simulink model "WaypointGuidanceDemo_students_model"  (R2024a)
settings: Solver=VariableStepAuto  StartTime=0.0  StopTime=t_final  MaxStep=deltaTMax  RelTol=1e-3
values from neighbouring files (symbols this model uses):
  flightRoute = FlightRoute(waypoints_ENU, isClosed)    [MAIN_WaypointGuidanceDemo_students.m]
  waypointRadius = 100    [MAIN_WaypointGuidanceDemo_students.m]
undefined symbols (not defined in the file or in its folder): magnitude
libraries: aerolibutil x2, spsEdgeDetectorLib x1, vrlib x1
settings Model: Creator=Christopher  LastModifiedBy=chris
settings SolverCC: AlgebraicLoopSolver=TrustRegion
settings DataIOCC: ReturnWorkspaceOutputs=off
settings DebuggingCC: UnconnectedInputMsg=warning  UnconnectedOutputMsg=warning  UnconnectedLineMsg=warning  ArithmeticOperatorsInVariantConditions=warning
settings ModelReferenceCC: EnableRefExpFcnMdlSchedulingChecks=on
settings SFSimCC: CustomCodeUndefinedFunction=UseInterfaceOnly
settings RTWCC: GPUComputeCapability=3.5  DLArmComputeVersion=19.05

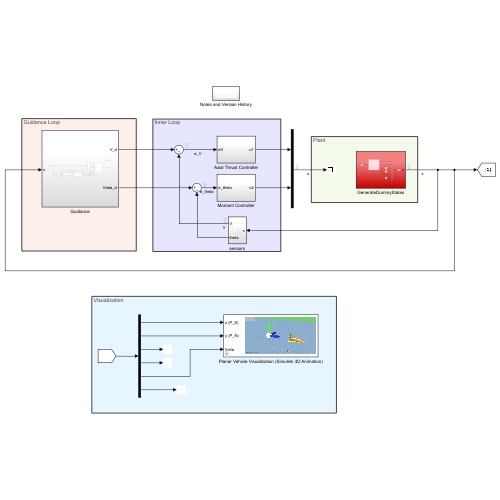
[thumbnail: Simulink's stored preview of the top-level diagram]
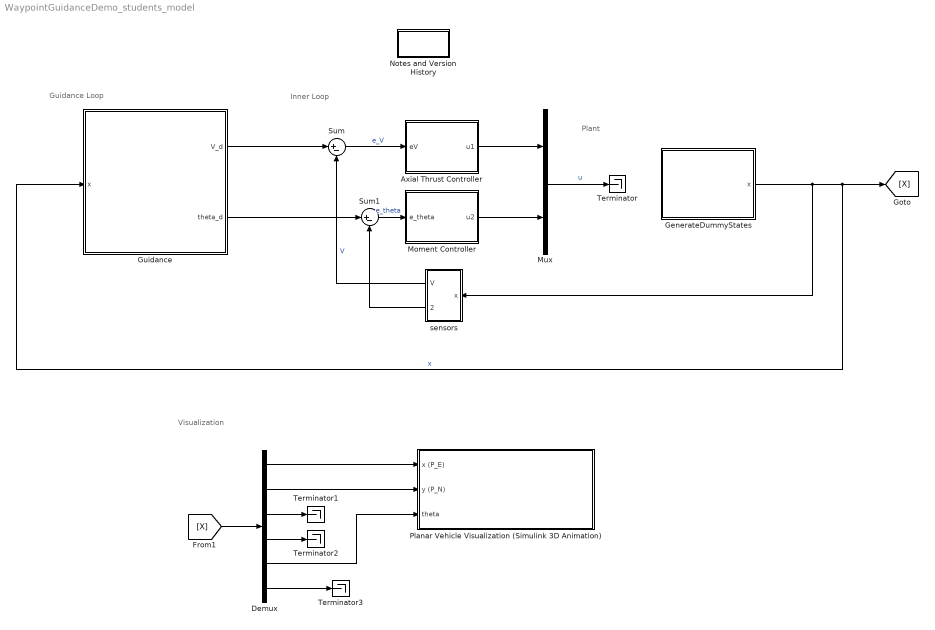
== system WaypointGuidanceDemo_students_model ==
  note: Plant
  note: Visualization
  note: Guidance Loop
  note: Inner Loop
  Axial Thrust Controller : Subsystem
  Demux : Demux  Outputs=6
  GenerateDummyStates : Subsystem
  Guidance : Subsystem
  Moment Controller : Subsystem
  Mux : Mux  Inputs=2
  Notes and Version History : Subsystem
  Planar Vehicle Visualization (Simulink 3D Animation) : Subsystem  mask{T_animate=1}
      mask prompts: T_animate "Time step for animation"
      mask help:
      | This is a visualization of the planar vehicle using the Simulink 3D Animation environment.
      |
      | Note: Simulink should open up the VRML sink and it should display the aircraft model in a separate window.  If this does not occur, you may need to look under the mask and through down through subsystems until you find the VR Sink block.  Double click on this block to open the animation window.
      |
      | Further note that Simulink may close the VRML sink the first time it is run (it may display a warning with verbiage about 'Virtual world has been closed from outside of Simulink.'.  If this occurs, simply repeat the procedure of looking under the mask and double clicking on the VR Sink.
      |
      | INPUTS:
      | -x: x-position (position east)
      | -y: y-position (position north)
      | -theta: heading angle (0 = pointing in +y (east) direction, positive counter-clockwise) (rad)
      |
      | Christopher Lum
      | lum@uw.edu
      mask Display: image('Simulink3Visualization.png')
  Sum : Sum  Inputs=|+-
  Sum1 : Sum  Inputs=|+-
  Terminator{,1..3} (4 alike) : Terminator
  sensors : Subsystem
  wires:
  Mux/1 -> Terminator/1  "u"
  Axial Thrust Controller/1(u1) -> Mux/1
  Moment Controller/1(u2) -> Mux/2
  sensors/2(theta) -> Sum1/2
  sensors/1(V) -> Sum/2  "V"
  Sum/1 -> Axial Thrust Controller/1(eV)  "e_V"
  Sum1/1 -> Moment Controller/1(e_theta)  "e_theta"
  [X] -> Demux/1
  Demux/1 -> Planar Vehicle Visualization (Simulink 3D Animation)/1(x (P_E))
  Demux/2 -> Planar Vehicle Visualization (Simulink 3D Animation)/2(y (P_N))
  Demux/3 -> Terminator1/1
  Demux/4 -> Terminator2/1
  Demux/6 -> Terminator3/1
  Demux/5 -> Planar Vehicle Visualization (Simulink 3D Animation)/3(theta)
  GenerateDummyStates/1(x) -> sensors/1(x), [X], Guidance/1(x)  "x"
  Guidance/1(V_d) -> Sum/1
  Guidance/2(theta_d) -> Sum1/1

== system WaypointGuidanceDemo_students_model/Axial Thrust Controller ==
  eV : Inport
  Ground : Ground
  Terminator : Terminator
  u1 : Outport  VectorParamsAs1DForOutWhenUnconnected=off
  wires:
  Ground/1 -> u1/1
  eV/1 -> Terminator/1

== system WaypointGuidanceDemo_students_model/GenerateDummyStates ==
  Clock : Clock
  Ground : Ground
  Ground1 : Ground
  Ground2 : Ground
  MATLAB Function : MATLAB Function  TreatAsAtomicUnit=on
  Mux : Mux  Inputs=6
  x : Outport
  wires:
  Mux/1 -> x/1
  Ground/1 -> Mux/3
  Ground1/1 -> Mux/4
  Ground2/1 -> Mux/6
  Clock/1 -> MATLAB Function/1(t)
  MATLAB Function/2(y) -> Mux/2
  MATLAB Function/1(x) -> Mux/1
  MATLAB Function/3(theta) -> Mux/5

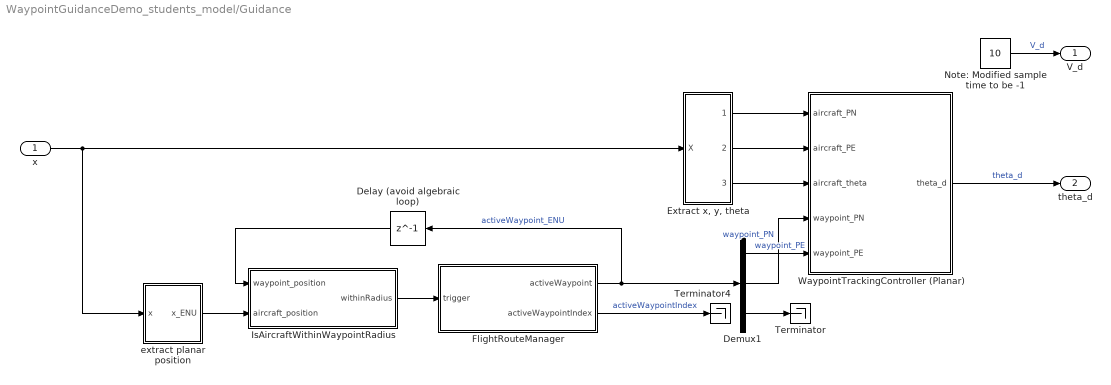
== system WaypointGuidanceDemo_students_model/Guidance ==
  x : Inport
  Delay (avoid algebraic loop) : Delay  DelayLength=1
  Demux1 : Demux  Outputs=3
  "Extract x, y, theta" : Subsystem
  FlightRouteManager : Subsystem  mask{waypoints=flightRoute.Points, isClosedRoute=on}
      mask prompts: waypoints "Waypoints (3xN matrix)"; isClosedRoute "Closed route"
      mask help:
      | Manages a flight route.  The flight route is a matrix of waypoints as a 3xN matrix.  This block outputs the coordinates and index of the active/current waypoint.
      |
      | When it is desired to increment the active waypoint index (for example the vehicle reaches the active/current waypoint), the 'trigger' signal should go from zero to any non-zero value to indicate this transition.  The increment of active waypoint will occur on this raising/falling edge.
      |
      | PARAMETERS:
      | -Waypoints: 3xN matrix describing the coordinates of each waypoint
      | -Closed route: checked = closed route implies that the active waypoint after the last waypoint is the first waypoint (wraps around), unchecked = open route and the active waypoint will remain at the last waypoint.
      |
      | INPUT:
      | -trigger: triggering signal
      |
      | OUTPUT:
      | -activeWaypoint:	3x1 coordinate of the active waypoint
      | -activeWaypointIndex:	active waypoint index
      |
      | Created by Christopher Lum
      | lum@uw.edu
  IsAircraftWithinWaypointRadius : Subsystem  mask{R=waypointRadius}
      mask prompts: R "Waypoint radius"
      mask help:
      | Simple logic to determine if a vehicle has reached within a certain radius of a waypoint.
      |
      | PARAMETERS:
      | -Waypoint radius: waypoint is reached when vehicle is within this distance of the waypoint
      |
      | INPUT:
      | -waypoint_position: 3 element vector describing the position of the waypoint
      | -aircraft_position: 3 element vector describing the position of the aircraft
      |
      | OUTPUT:
      | -withinRadius: boolean denoting if aircraft is within radius or not.
      |
      | Created by Christopher Lum
      | lum@uw.edu
      mask TypeOptions R: Constant/Value
  Note: Modified sample time to be -1 : Constant  Value=10  SampleTime=-1
  Terminator : Terminator
  Terminator4 : Terminator
  WaypointTrackingController (Planar) : Subsystem
      mask help:
      | Determine the heading angle the aircraft should have in order to be pointing towards the waypoint.
      |
      | PARAMETERS:
      | -None
      |
      | INPUT:
      | -aircraft_PN: position north of the aircraft
      | -aircraft_PE: position east of the aircraft
      | -aircraft_theta: heading angle of the aircraft (0 = pointing East, positive CCW)
      | -waypoint_PN: position north of the waypoint
      | -waypoint_PE: position east of the waypoint
      |
      | OUTPUT:
      | -theta_d: desired heading angle so aircraft is pointing towards waypoint
      |
      | Created by Christopher Lum
      | lum@uw.edu
  extract planar position : Subsystem
  V_d : Outport  VectorParamsAs1DForOutWhenUnconnected=off
  theta_d : Outport  Port=2  VectorParamsAs1DForOutWhenUnconnected=off
  wires:
  x/1 -> "Extract x, y, theta"/1(X), extract planar position/1(x)
  extract planar position/1(x_ENU) -> IsAircraftWithinWaypointRadius/2(aircraft_position)
  "Extract x, y, theta"/1(y = PN) -> WaypointTrackingController (Planar)/1(aircraft_PN)
  FlightRouteManager/2(activeWaypointIndex) -> Terminator4/1  "activeWaypointIndex"
  FlightRouteManager/1(activeWaypoint) -> Delay (avoid algebraic loop)/1, Demux1/1  "activeWaypoint_ENU"
  Demux1/1 -> WaypointTrackingController (Planar)/5(waypoint_PE)  "waypoint_PE"
  Demux1/3 -> Terminator/1
  IsAircraftWithinWaypointRadius/1(withinRadius) -> FlightRouteManager/1(trigger)
  Delay (avoid algebraic loop)/1 -> IsAircraftWithinWaypointRadius/1(waypoint_position)
  Demux1/2 -> WaypointTrackingController (Planar)/4(waypoint_PN)  "waypoint_PN"
  "Extract x, y, theta"/3(theta) -> WaypointTrackingController (Planar)/3(aircraft_theta)
  "Extract x, y, theta"/2(x = PE) -> WaypointTrackingController (Planar)/2(aircraft_PE)
  Note: Modified sample time to be -1/1 -> V_d/1  "V_d"
  WaypointTrackingController (Planar)/1(theta_d) -> theta_d/1  "theta_d"

== system WaypointGuidanceDemo_students_model/Moment Controller ==
  e_theta : Inport
  Ground : Ground
  Terminator : Terminator
  u2 : Outport  VectorParamsAs1DForOutWhenUnconnected=off
  wires:
  e_theta/1 -> Terminator/1
  Ground/1 -> u2/1

== system WaypointGuidanceDemo_students_model/Notes and Version History ==
  note: Skeleton code to show how to perform guidance and inner loop control with a planar vehicle.
      |
      | Christopher Lum
      | lum@uw.edu
      |
      | Version History
      | 06/04/19: Created from previous model
      | 06/05/19: Updated
      | 06/06/19: Adding Simulink 3D Animation visualization
      | 06/07/19: Added waypoint following.  Confirmed to work.
      | 04/04/21: Tested and confirmed to work after removing the wrapping of theta.  Rewired diagram
      | 05/20/21: Broke all links so this is usable by TA and students
      | 05/02/23: Fixed sample time of constant block to be -1 instead of inf
      | 02/15/25: Changed how signals are logged.  Added dummy state signals.  Moved to GitHub.

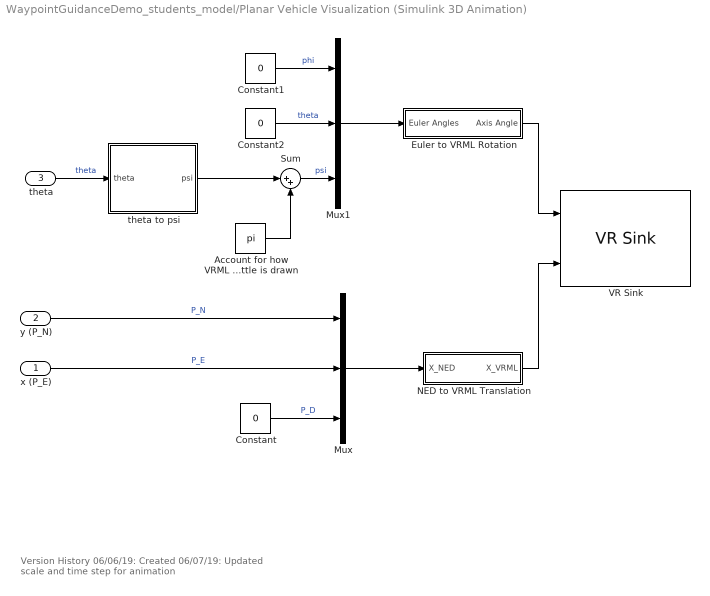
== system WaypointGuidanceDemo_students_model/Planar Vehicle Visualization (Simulink 3D Animation) ==
  note: Version History
      | 06/06/19: Created
      | 06/07/19: Updated scale and time step for animation
  x (P_E) : Inport
  y (P_N) : Inport  Port=2
  theta : Inport  Port=3
  Account for how VRML Shuttle is drawn : Constant  Value=pi
  Constant : Constant  Value=0
  Constant1 : Constant  Value=0
  Constant2 : Constant  Value=0
  Euler to VRML Rotation : Subsystem
      mask help:
      | Convert a set of Euler angles so it is suitable to be input to a VR Sink block for rotation.
      |
      | INPUT:
      | Euler: 3x1 vector of standard Euler zyx-rotation sequence [phi;theta;psi]
      |
      | OUTPUT:
      | Axis Angle: 4x1 vector of rotation to be used in VRML
      |
      | Created by Christopher Lum
      | lum@uw.edu
  Mux : Mux  Inputs=3
  Mux1 : Mux  Inputs=3
  NED to VRML Translation : Subsystem
      mask help:
      | Convert a position so it is suitable to be input to a VR Sink block for tranlation/position.
      |
      | INPUT:
      | X_NED: 3x1 vector of position in [P_N; P_E; P_D]
      |
      | OUTPUT:
      | X_VRML: 3x1 vector of position in [P_N; P_U; P_E]
      |
      | Created by Christopher Lum
      | lum@uw.edu
  Sum : Sum  Inputs=|++
  VR Sink : vrlib/VR Sink  InstantiateOnLoad=on  SampleTime=T_animate  ViewEnable=on  RemoteChange=off  RemoteView=off  FieldsWritten=Shuttle.rotation.4.1.1.double#Shuttle.translation.3.1.1.double  WorldFileName=PugetSound.wrl  AutoView=on  VideoDimensions=[]  AllowVariableSize=off  FigureProperties="{'Position', 'Name', 'Viewpoint', 'CameraBound', 'CameraDirection', 'CameraPosition', 'CameraUpVector', 'ZoomFactor', 'Antialiasing', 'Headlight', 'Lighting', 'Sound', 'StatusBar', 'Stereo3D', 'Stereo3DCameraOffset', 'Stereo3DHIT', 'ToolBar', 'Textures', 'Transparency', 'Triad', 'Wireframe', 'NavZones', 'NavMode', 'NavSpeed', 'CaptureFileFormat', 'CaptureFileName', 'Record2DCompressMethod', 'Record2DCompressQuality', 'Record2D', 'Record2DFileName', 'Record2DFPS', 'NavPanel'; [5.0000000000000000e+00   9.2000000000000000e+01   1.0470000000000000e+03   6.8100000000000000e+02], '', 'TopView', 'on', [0.0000000000000000e+00   0.0000000000000000e+00  -1.0000000000000000e+00], [0.0000000000000000e+00   0.0000000000000000e+00   0.0000000000000000e+00], [0.0000000000000000e+00   1.0000000000000000e+00   0.0000000000000000e+00], [1.0000000000000000e+00], 'on', 'on', 'on', 'on', 'on', 'off', [1.0000000149011612e-01], [0.0000000000000000e+00], 'on', 'on', 'on', 'none', 'off', 'off', 'fly', 'normal', 'tif', '%f_anim_%n.tif', 'auto', [7.5000000000000000e+01], 'off', '%f_anim_%n.avi', 'auto', 'halfbar'}"
  theta to psi : Subsystem
  wires:
  Constant1/1 -> Mux1/1  "phi"
  Constant/1 -> Mux/3  "P_D"
  Mux/1 -> NED to VRML Translation/1(X_NED)
  Mux1/1 -> Euler to VRML Rotation/1(Euler Angles)
  NED to VRML Translation/1(X_VRML) -> VR Sink/2
  x (P_E)/1 -> Mux/2  "P_E"
  theta to psi/1(psi) -> Sum/1
  Account for how VRML Shuttle is drawn/1 -> Sum/2
  Constant2/1 -> Mux1/2  "theta"
  Sum/1 -> Mux1/3  "psi"
  theta/1 -> theta to psi/1(theta)  "theta"
  y (P_N)/1 -> Mux/1  "P_N"
  Euler to VRML Rotation/1(Axis Angle) -> VR Sink/1

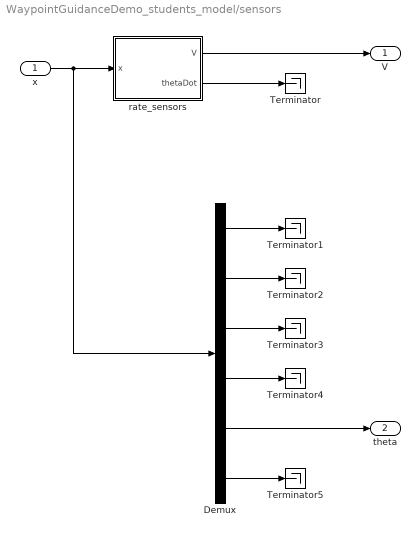
== system WaypointGuidanceDemo_students_model/sensors ==
  x : Inport
  Demux : Demux  Outputs=6
  Terminator{,1..5} (6 alike) : Terminator
  rate_sensors : Subsystem
      mask help:
      | Models rate sensors which measure the translational and rotational velocity of the vehicle.
      |
      | INPUTS:
      | -x: 6x1 state vector
      |
      | OUTPUTS:
      | -V: scalar representing planar velocity (m/s)
      | -thetaDot: scalar representing rotational velocity (rad/s)
      |
      | Created by Christopher Lum
      | lum@uw.edu
  V : Outport  VectorParamsAs1DForOutWhenUnconnected=off
  theta : Outport  Port=2  VectorParamsAs1DForOutWhenUnconnected=off
  wires:
  x/1 -> Demux/1, rate_sensors/1(x)
  rate_sensors/1(V) -> V/1
  Demux/5 -> theta/1
  rate_sensors/2(thetaDot) -> Terminator/1
  Demux/1 -> Terminator1/1
  Demux/2 -> Terminator2/1
  Demux/3 -> Terminator3/1
  Demux/4 -> Terminator4/1
  Demux/6 -> Terminator5/1

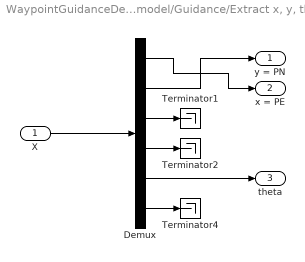
== system WaypointGuidanceDemo_students_model/Guidance/Extract x, y, theta ==
  X : Inport
  Demux : Demux  Outputs=6
  Terminator1 : Terminator
  Terminator2 : Terminator
  Terminator4 : Terminator
  y = PN : Outport  VectorParamsAs1DForOutWhenUnconnected=off
  x = PE : Outport  Port=2  VectorParamsAs1DForOutWhenUnconnected=off
  theta : Outport  Port=3  VectorParamsAs1DForOutWhenUnconnected=off
  wires:
  Demux/5 -> theta/1
  Demux/4 -> Terminator2/1
  Demux/3 -> Terminator1/1
  Demux/6 -> Terminator4/1
  X/1 -> Demux/1
  Demux/2 -> y = PN/1
  Demux/1 -> x = PE/1

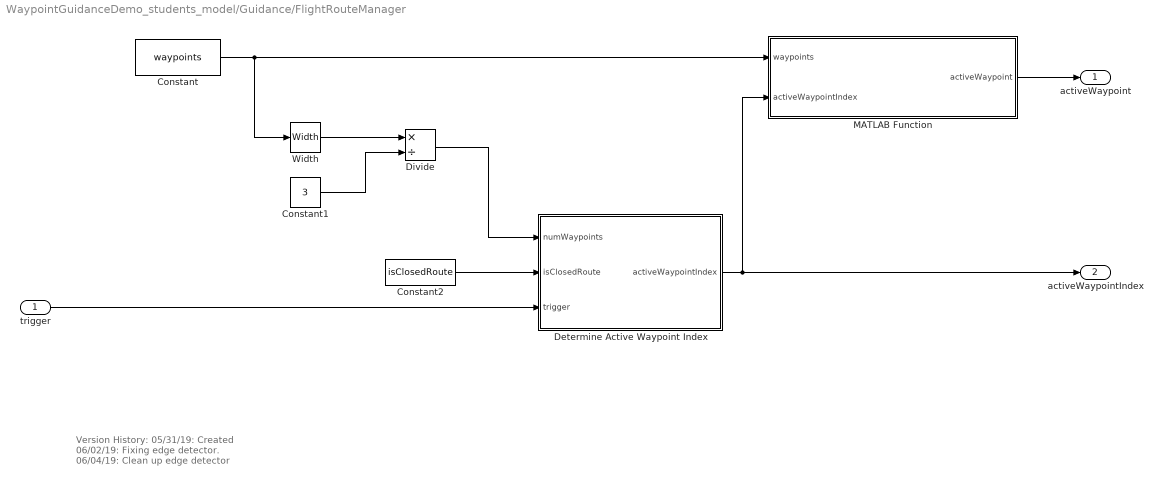
== system WaypointGuidanceDemo_students_model/Guidance/FlightRouteManager ==
  note: Version History:
      | 05/31/19: Created
      | 06/02/19: Fixing edge detector.
      | 06/04/19: Clean up edge detector
  trigger : Inport
  Constant : Constant  Value=waypoints
  Constant1 : Constant  Value=3
  Constant2 : Constant  Value=isClosedRoute  OutDataTypeStr=boolean
  Determine Active Waypoint Index : Subsystem
  Divide : Product  Inputs=*/
  MATLAB Function : MATLAB Function  TreatAsAtomicUnit=on
  Width : Width
  activeWaypoint : Outport  VectorParamsAs1DForOutWhenUnconnected=off
  activeWaypointIndex : Outport  Port=2  VectorParamsAs1DForOutWhenUnconnected=off
  wires:
  Constant2/1 -> Determine Active Waypoint Index/2(isClosedRoute)
  trigger/1 -> Determine Active Waypoint Index/3(trigger)
  Divide/1 -> Determine Active Waypoint Index/1(numWaypoints)
  Constant1/1 -> Divide/2
  Width/1 -> Divide/1
  Determine Active Waypoint Index/1(activeWaypointIndex) -> activeWaypointIndex/1, MATLAB Function/2(activeWaypointIndex)
  MATLAB Function/1(activeWaypoint) -> activeWaypoint/1
  Constant/1 -> MATLAB Function/1(waypoints), Width/1

== system WaypointGuidanceDemo_students_model/Guidance/IsAircraftWithinWaypointRadius ==
  note: Version History
      | 06/04/19: Created
  waypoint_position : Inport
  aircraft_position : Inport  Port=2
  Constant : Constant  Value=R
  Relational Operator : RelationalOperator  Operator=<=  OutDataTypeStr=boolean  RndMeth=Simplest  InputSameDT=off
  Sum : Sum  Inputs=|+-
  vector_2_norm : Subsystem
      mask help:
      | Compute the 2-norm of a 3 dimensional vector
      |
      |     y = norm(x) = sqrt(x(1)^2 + x(2)^2 + x(3)^2)
      |
      | INPUT:  x:  3x1 vector
      |
      | OUTPUT: norm(x):    2-norm of x
      |
      | VALIDATION: none
  withinRadius : Outport  VectorParamsAs1DForOutWhenUnconnected=off
  wires:
  Relational Operator/1 -> withinRadius/1
  Constant/1 -> Relational Operator/2
  vector_2_norm/1(norm(x)) -> Relational Operator/1
  Sum/1 -> vector_2_norm/1(x)
  aircraft_position/1 -> Sum/2
  waypoint_position/1 -> Sum/1

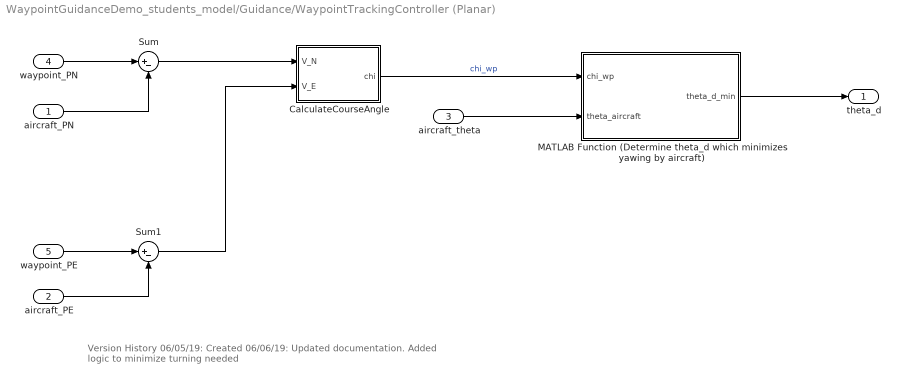
== system WaypointGuidanceDemo_students_model/Guidance/WaypointTrackingController (Planar) ==
  note: Version History
      | 06/05/19: Created
      | 06/06/19: Updated documentation.  Added logic to minimize turning needed
  aircraft_PN : Inport
  aircraft_PE : Inport  Port=2
  aircraft_theta : Inport  Port=3
  waypoint_PN : Inport  Port=4
  waypoint_PE : Inport  Port=5
  CalculateCourseAngle : Subsystem
      mask help:
      | Calculate the course angle (chie) given the north velocity (V_N) and east velocity (V_E).
      |
      | A heading of chi = 0 implies a course of directly north.
      |
      | The units of V_N and V_E must be teh same.  chi is restricted to the range of [0, 2*pi).
      |
      | INPUTS:
      | -V_N: North velocity
      | -V_E: East velocity
      |
      | OUTPUTS:
      | -chi: course angle in range of [0, 2*pi) (radians)
      |
      | Created by Christopher Lum
      | lum@uw.edu
  MATLAB Function (Determine theta_d which minimizes yawing by aircraft) : MATLAB Function  TreatAsAtomicUnit=on
  Sum : Sum  Inputs=|+-
  Sum1 : Sum  Inputs=|+-
  theta_d : Outport  VectorParamsAs1DForOutWhenUnconnected=off
  wires:
  MATLAB Function (Determine theta_d which minimizes yawing by aircraft)/1(theta_d_min) -> theta_d/1
  aircraft_theta/1 -> MATLAB Function (Determine theta_d which minimizes yawing by aircraft)/2(theta_aircraft)
  CalculateCourseAngle/1(chi) -> MATLAB Function (Determine theta_d which minimizes yawing by aircraft)/1(chi_wp)  "chi_wp"
  Sum1/1 -> CalculateCourseAngle/2(V_E)
  Sum/1 -> CalculateCourseAngle/1(V_N)
  aircraft_PE/1 -> Sum1/2
  waypoint_PE/1 -> Sum1/1
  aircraft_PN/1 -> Sum/2
  waypoint_PN/1 -> Sum/1

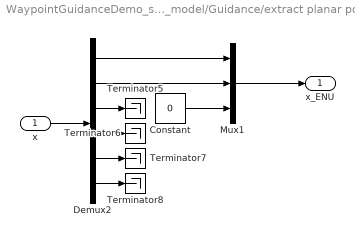
== system WaypointGuidanceDemo_students_model/Guidance/extract planar position ==
  x : Inport
  Constant : Constant  Value=0
  Demux2 : Demux  Outputs=6
  Mux1 : Mux  Inputs=3
  Terminator{5..8} (4 alike) : Terminator
  x_ENU : Outport  VectorParamsAs1DForOutWhenUnconnected=off
  wires:
  Demux2/4 -> Terminator6/1
  Mux1/1 -> x_ENU/1
  Demux2/3 -> Terminator5/1
  x/1 -> Demux2/1
  Constant/1 -> Mux1/3
  Demux2/2 -> Mux1/2
  Demux2/5 -> Terminator7/1
  Demux2/6 -> Terminator8/1
  Demux2/1 -> Mux1/1

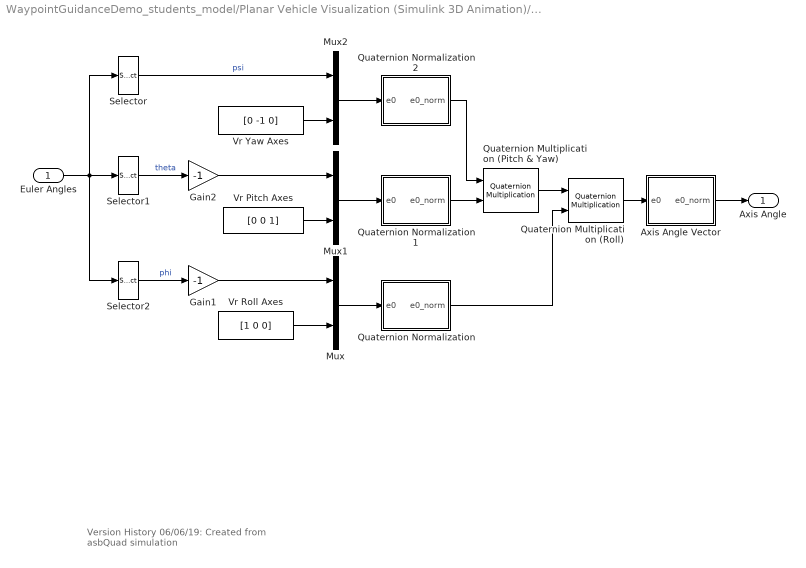
== system WaypointGuidanceDemo_students_model/Planar Vehicle Visualization (Simulink 3D Animation)/Euler to VRML Rotation ==
  note: Version History
      | 06/06/19: Created from asbQuad simulation
  Euler Angles : Inport
  Axis Angle Vector : Subsystem
  Gain1 : Gain  Gain=-1
  Gain2 : Gain  Gain=-1
  Mux : Mux  Inputs=2
  Mux1 : Mux  Inputs=2
  Mux2 : Mux  Inputs=2
  Quaternion Multiplication (Pitch & Yaw) : aerolibutil/Quaternion Multiplication
  Quaternion Multiplication (Roll) : aerolibutil/Quaternion Multiplication
  Quaternion Normalization : Subsystem
  Quaternion Normalization1 : Subsystem
  Quaternion Normalization2 : Subsystem
  Selector : Selector  InputPortWidth=3  IndexOptions=Index vector (dialog)  Indices=[3]  OutputSizes=1
  Selector1 : Selector  InputPortWidth=3  IndexOptions=Index vector (dialog)  Indices=[2]  OutputSizes=1
  Selector2 : Selector  InputPortWidth=3  IndexOptions=Index vector (dialog)  Indices=[1]  OutputSizes=1
  Vr Pitch Axes : Constant  Value=[0 0 1]
  Vr Roll Axes : Constant  Value=[1 0 0]
  Vr Yaw Axes : Constant  Value=[0 -1 0]
  Axis Angle : Outport  VectorParamsAs1DForOutWhenUnconnected=off
  wires:
  Gain2/1 -> Mux1/1
  Gain1/1 -> Mux/1
  Euler Angles/1 -> Selector1/1, Selector/1, Selector2/1
  Quaternion Multiplication (Pitch & Yaw)/1 -> Quaternion Multiplication (Roll)/1
  Vr Roll Axes/1 -> Mux/2
  Selector2/1 -> Gain1/1  "phi"
  Vr Pitch Axes/1 -> Mux1/2
  Selector1/1 -> Gain2/1  "theta"
  Vr Yaw Axes/1 -> Mux2/2
  Selector/1 -> Mux2/1  "psi"
  Mux/1 -> Quaternion Normalization/1(e0)
  Mux1/1 -> Quaternion Normalization1/1(e0)
  Mux2/1 -> Quaternion Normalization2/1(e0)
  Quaternion Normalization1/1(e0_norm) -> Quaternion Multiplication (Pitch & Yaw)/2
  Quaternion Normalization2/1(e0_norm) -> Quaternion Multiplication (Pitch & Yaw)/1
  Quaternion Normalization/1(e0_norm) -> Quaternion Multiplication (Roll)/2
  Axis Angle Vector/1(e0_norm) -> Axis Angle/1
  Quaternion Multiplication (Roll)/1 -> Axis Angle Vector/1(e0)

== system WaypointGuidanceDemo_students_model/Planar Vehicle Visualization (Simulink 3D Animation)/NED to VRML Translation ==
  note: Version History
      | 06/05/19: Created
  X_NED : Inport
  Demux : Demux  Outputs=3
      settings: DisplayOption=none
  Mux : Mux  Inputs=3
  rad-->deg1 : Gain  Gain=-1  SaturateOnIntegerOverflow=on  OutDataTypeStr=Inherit: Same as input  ParamDataTypeStr=Inherit: Same as input
  X_VRML : Outport  VectorParamsAs1DForOutWhenUnconnected=off
  wires:
  X_NED/1 -> Demux/1
  Mux/1 -> X_VRML/1
  Demux/3 -> rad-->deg1/1
  Demux/2 -> Mux/3
  Demux/1 -> Mux/1
  rad-->deg1/1 -> Mux/2

== system WaypointGuidanceDemo_students_model/Planar Vehicle Visualization (Simulink 3D Animation)/theta to psi ==
  theta : Inport
  Constant : Constant  Value=pi/2
  Sum : Sum  Inputs=|-+
  psi : Outport  VectorParamsAs1DForOutWhenUnconnected=off
  wires:
  Sum/1 -> psi/1
  Constant/1 -> Sum/2
  theta/1 -> Sum/1

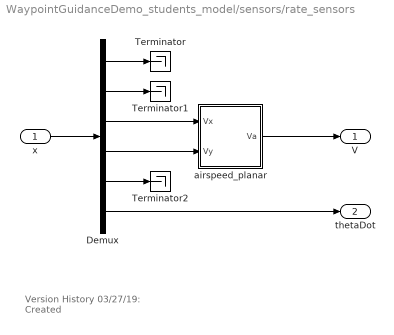
== system WaypointGuidanceDemo_students_model/sensors/rate_sensors ==
  note: Version History
      | 03/27/19: Created
  x : Inport
  Demux : Demux  Outputs=6
  Terminator : Terminator
  Terminator1 : Terminator
  Terminator2 : Terminator
  airspeed_planar : Subsystem
      mask help:
      | Calculates the planar airsppeed.
      |
      | INPUTS
      | -Vx: X comopoent of velocity
      | -Vy: Y component of velocity
      |
      | OUTPUTS
      | -Va: Scalar of the airspeed.
      |
      | Created by Christopher Lum
      | lum@uw.edu
  V : Outport  VectorParamsAs1DForOutWhenUnconnected=off
  thetaDot : Outport  Port=2  VectorParamsAs1DForOutWhenUnconnected=off
  wires:
  Demux/6 -> thetaDot/1
  airspeed_planar/1(Va) -> V/1
  Demux/5 -> Terminator2/1
  Demux/4 -> airspeed_planar/2(Vy)
  Demux/3 -> airspeed_planar/1(Vx)
  Demux/2 -> Terminator1/1
  Demux/1 -> Terminator/1
  x/1 -> Demux/1

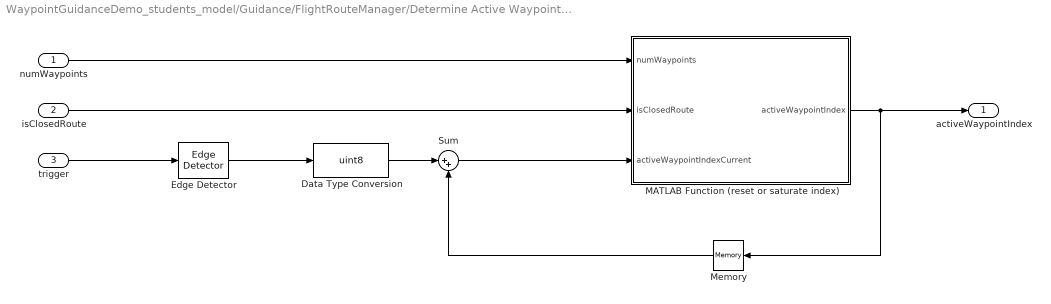
== system WaypointGuidanceDemo_students_model/Guidance/FlightRouteManager/Determine Active Waypoint Index ==
  numWaypoints : Inport
  isClosedRoute : Inport  Port=2
  trigger : Inport  Port=3
  Data Type Conversion : DataTypeConversion  OutDataTypeStr=uint8  SaturateOnIntegerOverflow=off  RndMeth=Floor
  Edge Detector : spsEdgeDetectorLib/Edge Detector  model=Rising  ic=0  Ts=0
      settings: LibrarySourceBlock=sps_lib/Control/Edge Detector
  MATLAB Function (reset or saturate index) : MATLAB Function  TreatAsAtomicUnit=on
  Memory : Memory  InitialCondition=1
  Sum : Sum  Inputs=|++
  activeWaypointIndex : Outport  VectorParamsAs1DForOutWhenUnconnected=off
  wires:
  isClosedRoute/1 -> MATLAB Function (reset or saturate index)/2(isClosedRoute)
  trigger/1 -> Edge Detector/1
  MATLAB Function (reset or saturate index)/1(activeWaypointIndex) -> activeWaypointIndex/1, Memory/1
  numWaypoints/1 -> MATLAB Function (reset or saturate index)/1(numWaypoints)
  Sum/1 -> MATLAB Function (reset or saturate index)/3(activeWaypointIndexCurrent)
  Memory/1 -> Sum/2
  Edge Detector/1 -> Data Type Conversion/1
  Data Type Conversion/1 -> Sum/1

== system WaypointGuidanceDemo_students_model/Guidance/IsAircraftWithinWaypointRadius/vector_2_norm ==
  x : Inport
  Demux : Demux  Outputs=3
  Math Function : Math  Operator=magnitude^2  SignedPower=on
  Sqrt : Sqrt
  Sum : Sum  Inputs=+|+|+
  norm(x) : Outport  VectorParamsAs1DForOutWhenUnconnected=off
  wires:
  x/1 -> Math Function/1
  Math Function/1 -> Demux/1
  Demux/1 -> Sum/1
  Demux/2 -> Sum/2
  Demux/3 -> Sum/3
  Sum/1 -> Sqrt/1
  Sqrt/1 -> norm(x)/1

== system WaypointGuidanceDemo_students_model/Guidance/WaypointTrackingController (Planar)/CalculateCourseAngle ==
  note: Version History
      | 06/05/19: Created
  V_N : Inport
  V_E : Inport  Port=2
  Constant : Constant  Value=pi/2
  Sum : Sum  Inputs=|+-
  Trigonometric Function : Trigonometry  Operator=atan2
  "[0,2*pi) Bound" : Subsystem  Description=|
      | Version History  
      |                  
      | 05/??/05: Created
      mask help:
      | Converts input angle to it equivalent in the range [0,2*pi).
      |
      | Inputs:		In: input angle (rad)
      | Outputs:	Out (bounded): bounded angle in range [0,2*pi).
      |
      | Created by Christopher Lum
      | lum@u.washington.edu
      |
      | Original Block concept from Aerosim Blockset by Unmanned Dynamics.  www.u-dynamics.com
  chi : Outport  VectorParamsAs1DForOutWhenUnconnected=off
  wires:
  Sum/1 -> "[0,2*pi) Bound"/1(in)
  Constant/1 -> Sum/1
  Trigonometric Function/1 -> Sum/2  "theta"
  "[0,2*pi) Bound"/1(out (bounded)) -> chi/1
  V_E/1 -> Trigonometric Function/2
  V_N/1 -> Trigonometric Function/1

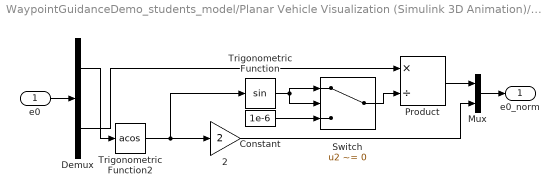
== system WaypointGuidanceDemo_students_model/Planar Vehicle Visualization (Simulink 3D Animation)/Euler to VRML Rotation/Axis Angle Vector ==
  e0 : Inport
  2 : Gain  Gain=2  SaturateOnIntegerOverflow=on  OutDataTypeStr=Inherit: Same as input  ParamDataTypeStr=Inherit: Same as input
  Constant : Constant  Value=1e-6
  Demux : Demux  Outputs=[1 3 ]
      settings: DisplayOption=none
  Mux : Mux  Inputs=2
  Product : Product  Inputs=*/  InputSameDT=on  SaturateOnIntegerOverflow=on  OutDataTypeStr=Inherit: Same as first input
  Switch : Switch  Criteria=u2 ~= 0  SaturateOnIntegerOverflow=off  InputSameDT=off
  Trigonometric Function : Trigonometry
  Trigonometric Function2 : Trigonometry  Operator=acos
  e0_norm : Outport  VectorParamsAs1DForOutWhenUnconnected=off
  wires:
  Switch/1 -> Product/2
  Constant/1 -> Switch/3
  e0/1 -> Demux/1
  Trigonometric Function2/1 -> 2/1, Trigonometric Function/1
  Trigonometric Function/1 -> Switch/2, Switch/1
  2/1 -> Mux/2
  Product/1 -> Mux/1
  Mux/1 -> e0_norm/1
  Demux/2 -> Product/1
  Demux/1 -> Trigonometric Function2/1

== system WaypointGuidanceDemo_students_model/Planar Vehicle Visualization (Simulink 3D Animation)/Euler to VRML Rotation/Quaternion Normalization ==
  e0 : Inport
  1/2 : Gain  Gain=1/2  SaturateOnIntegerOverflow=on  OutDataTypeStr=Inherit: Same as input  ParamDataTypeStr=Inherit: Same as input
  Demux : Demux  Outputs=[1 3]
      settings: DisplayOption=none
  Mux : Mux  Inputs=2
  Product : Product  InputSameDT=on  SaturateOnIntegerOverflow=on  OutDataTypeStr=Inherit: Same as first input
  Trigonometric Function : Trigonometry
  Trigonometric Function1 : Trigonometry  Operator=cos
  e0_norm : Outport  VectorParamsAs1DForOutWhenUnconnected=off
  wires:
  e0/1 -> Demux/1
  1/2/1 -> Trigonometric Function/1, Trigonometric Function1/1
  Trigonometric Function/1 -> Product/1
  Product/1 -> Mux/2
  Mux/1 -> e0_norm/1
  Demux/1 -> 1/2/1
  Demux/2 -> Product/2
  Trigonometric Function1/1 -> Mux/1

== system WaypointGuidanceDemo_students_model/Planar Vehicle Visualization (Simulink 3D Animation)/Euler to VRML Rotation/Quaternion Normalization1 ==
  e0 : Inport
  1/2 : Gain  Gain=1/2  SaturateOnIntegerOverflow=on  OutDataTypeStr=Inherit: Same as input  ParamDataTypeStr=Inherit: Same as input
  Demux : Demux  Outputs=[1 3]
      settings: DisplayOption=none
  Mux : Mux  Inputs=2
  Product : Product  InputSameDT=on  SaturateOnIntegerOverflow=on  OutDataTypeStr=Inherit: Same as first input
  Trigonometric Function : Trigonometry
  Trigonometric Function1 : Trigonometry  Operator=cos
  e0_norm : Outport  VectorParamsAs1DForOutWhenUnconnected=off
  wires:
  Trigonometric Function1/1 -> Mux/1
  Demux/2 -> Product/2
  Demux/1 -> 1/2/1
  Mux/1 -> e0_norm/1
  Product/1 -> Mux/2
  Trigonometric Function/1 -> Product/1
  1/2/1 -> Trigonometric Function1/1, Trigonometric Function/1
  e0/1 -> Demux/1

== system WaypointGuidanceDemo_students_model/Planar Vehicle Visualization (Simulink 3D Animation)/Euler to VRML Rotation/Quaternion Normalization2 ==
  e0 : Inport
  1/2 : Gain  Gain=1/2  SaturateOnIntegerOverflow=on  OutDataTypeStr=Inherit: Same as input  ParamDataTypeStr=Inherit: Same as input
  Demux : Demux  Outputs=[1 3]
      settings: DisplayOption=none
  Mux : Mux  Inputs=2
  Product : Product  InputSameDT=on  SaturateOnIntegerOverflow=on  OutDataTypeStr=Inherit: Same as first input
  Trigonometric Function : Trigonometry
  Trigonometric Function1 : Trigonometry  Operator=cos
  e0_norm : Outport  VectorParamsAs1DForOutWhenUnconnected=off
  wires:
  e0/1 -> Demux/1
  1/2/1 -> Trigonometric Function/1, Trigonometric Function1/1
  Trigonometric Function/1 -> Product/1
  Product/1 -> Mux/2
  Mux/1 -> e0_norm/1
  Demux/1 -> 1/2/1
  Demux/2 -> Product/2
  Trigonometric Function1/1 -> Mux/1

== system WaypointGuidanceDemo_students_model/sensors/rate_sensors/airspeed_planar ==
  note: Version History
      | 03/26/19: Created
  Vx : Inport
  Vy : Inport  Port=2
  Math Function : Math  Operator=magnitude^2  SignedPower=on
  Math Function1 : Math  Operator=magnitude^2  SignedPower=on
  Sqrt : Sqrt
  Sum : Sum
  Va : Outport  VectorParamsAs1DForOutWhenUnconnected=off
  wires:
  Vy/1 -> Math Function1/1
  Math Function1/1 -> Sum/2
  Vx/1 -> Math Function/1
  Sqrt/1 -> Va/1
  Sum/1 -> Sqrt/1
  Math Function/1 -> Sum/1

== system WaypointGuidanceDemo_students_model/Guidance/WaypointTrackingController (Planar)/CalculateCourseAngle/[0,2*pi) Bound ==
  in : Inport
  Constant : Constant  Value=2*pi
  Math Function : Math  Operator=mod  SignedPower=on
  out (bounded) : Outport  VectorParamsAs1DForOutWhenUnconnected=off
  wires:
  Constant/1 -> Math Function/2
  Math Function/1 -> out (bounded)/1
  in/1 -> Math Function/1

== matlab function WaypointGuidanceDemo_students_model/Guidance/FlightRouteManager/MATLAB Function ==
  data: waypoints input; activeWaypoint output; activeWaypointIndex input
function activeWaypoint = fcn(waypoints, activeWaypointIndex)

%Create a FlightRoute object
flightRoute = FlightRoute(waypoints);

activeWaypoint = flightRoute.GetPoint(activeWaypointIndex);

== matlab function WaypointGuidanceDemo_students_model/Guidance/WaypointTrackingController (Planar)/MATLAB Function (Determine theta_d which minimizes yawing by aircraft) ==
  data: chi_wp input; theta_d_min output; theta_aircraft input
function theta_d_min  = fcn(chi_wp, theta_aircraft)

%convert chi to theta
theta_d = pi/2 - chi_wp;

%Determine if we need to add or subtract 2*pi to minimize required turning
theta_d_p2p = theta_d + 2*pi;
theta_d_m2p = theta_d - 2*pi;

%which yields the least error between the current aircraft theta
e_theta = theta_d - theta_aircraft;
e_theta_p2p = theta_d_p2p - theta_aircraft;
e_theta_m2p = theta_d_m2p - theta_aircraft;

[~,index] = min(abs([e_theta e_theta_p2p e_theta_m2p]));

switch index
    case 1
        %theta_d is best
        theta_d_min = theta_d;
        
    case 2
        %theta_d_p2p is best
        theta_d_min = theta_d_p2p;
        
    case 3
        %theta_d_m2p is best
        theta_d_min = e_theta_m2p;
        
    otherwise
        error('Unexpected error')
end

== matlab function WaypointGuidanceDemo_students_model/GenerateDummyStates/MATLAB Function ==
  data: x output; t input; y output; theta output
function [x,y,theta] = fcn(t)

a = 1500;
b = 750;

x = a*cos(2*pi*t/600);
y = b*sin(2*pi*t/600);
theta = 8*pi*t/600;

== matlab function WaypointGuidanceDemo_students_model/Guidance/FlightRouteManager/Determine Active Waypoint Index/MATLAB Function (reset or saturate index) ==
  data: numWaypoints input; isClosedRoute input; activeWaypointIndex output; activeWaypointIndexCurrent input
function activeWaypointIndex = fcn(numWaypoints, isClosedRoute, activeWaypointIndexCurrent)

%Saturate at maximum limit
if(activeWaypointIndexCurrent > numWaypoints)
    if(isClosedRoute)
        %Closed route: restart at waypoint 1
        activeWaypointIndex = 1;
    else
        %Open route: staturate at last waypoint.
        activeWaypointIndex = numWaypoints;
    end
    
else
    activeWaypointIndex = activeWaypointIndexCurrent;
    
end
